simulink model "M4B11_modified_AGC_PI"  (R2025a)
settings: Solver=VariableStepAuto  StartTime=0.0  StopTime=100  RelTol=1e-3
InitFcn:
  | clear;
  | load('parameterinit.mat');
  | set_param('M4B11_modified_AGC_PI/Python2Sim','value','[0 0 0 0 0 0 0 0]');
  | acom=100;
  | bcom=50;
  | lam=100;
values from neighbouring files (symbols this model uses):
  ACgirdinit =     [datainit.mat]    (also in parameterinit.mat)
  AVm0 = [11.3576294988 11.3576294988]    [datainit.mat]    (also in parameterinit.mat)
  commun = [1 1 1 0]    [datainit.mat]    (also in initAll.m = [1,1,1,0]; parameterinit.mat)
  DataDelay = [0  0; 0  0; 0  0; 0  0]    [datainit.mat]    (also in initAll.m = 0.0*DataDelay; parameterinit.mat)
  ESinit =     [datainit.mat]    (also in parameterinit.mat)
  fB = 50    [datainit.mat]    (also in initAll.m; parameterinit.mat)
  Geninit =     [datainit.mat]    (also in initAll.m = Generator_init(opdata,SynMach_in_gidx); parameterinit.mat)
  SgridB = 100    [datainit.mat]    (also in initAll.m = resultsac.baseMVA; parameterinit.mat)
  wB = 314.159265359    [datainit.mat]    (also in initAll.m; parameterinit.mat)
  Windinit =     [datainit.mat]    (also in parameterinit.mat)
undefined symbols (not defined in the file or in its folder): c1, c2, c3, c4, c5, c6, cp_nom, lambda_nom, P_wind_base, Pelec_base, Pnom
libraries: spsBistableLib x9, slpidlib x2, simulink_extras x2
(part 5 of 6)

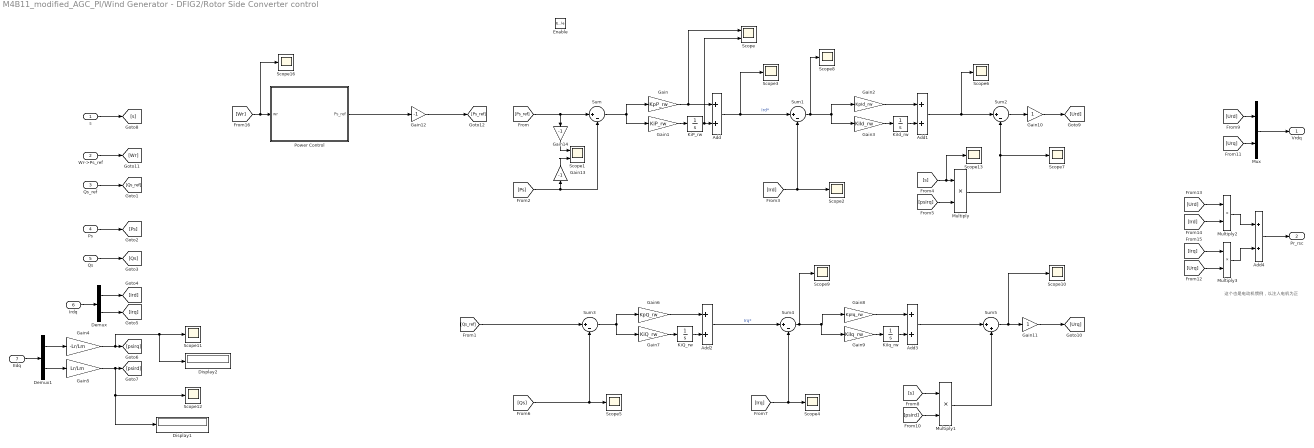
== system M4B11_modified_AGC_PI/Wind Generator - DFIG2/Rotor Side Converter control ==
  note: 这个也是电动机惯例，以注入电机为正
  s : Inport
  Wr->Ps_ref : Inport  Port=2
  Qs_ref : Inport  Port=3
  Ps : Inport  Port=4
  Qs : Inport  Port=5
  Irdq : Inport  Port=6
  Edq : Inport  Port=7
  Enable : EnablePort
  Add{,1..4} (5 alike) : Sum
  Demux : Demux  Outputs=2
  Demux1 : Demux  Outputs=2
  Display1 : Display
  Display2 : Display
  Gain : Gain  Gain=KpP_rw
  Gain1 : Gain  Gain=KiP_rw
  Gain10 : Gain
  Gain11 : Gain
  Gain12 : Gain  Gain=-1
  Gain13 : Gain  Gain=-1
  Gain14 : Gain  Gain=-1
  Gain2 : Gain  Gain=KpId_rw
  Gain3 : Gain  Gain=KiId_rw
  Gain4 : Gain  Gain=-Lr/Lm
  Gain5 : Gain  Gain=Lr/Lm
  Gain6 : Gain  Gain=KpQ_rw
  Gain7 : Gain  Gain=KiQ_rw
  Gain8 : Gain  Gain=KpIq_rw
  Gain9 : Gain  Gain=KiIq_rw
  KiId_rw : Integrator
  KiIq_rw : Integrator
  KiP_rw : Integrator  InitialCondition=Ird_ref
  KiQ_rw : Integrator  InitialCondition=Irq_ref
  Multiply{,1..3} (4 alike) : Product
  Mux : Mux  Inputs=2
  Power Control : Subsystem
  Scope : Scope  NumInputPorts=2
      settings: ActiveDisplayYMinimum=-0.15787  ActiveDisplayYMaximum=1.4048
  Scope1 : Scope  NumInputPorts=2
      settings: ActiveDisplayYMinimum=0.941157  ActiveDisplayYMaximum=0.94124  DataLoggingVariableName=ScopeData2
  Scope{2..13,16} (13 alike) : Scope
      Scope10 settings: ActiveDisplayYMinimum=-0.02713  ActiveDisplayYMaximum=0.00724  DataLoggingVariableName=ScopeData10
      Scope11 settings: DataLoggingVariableName=ScopeData13
      Scope12 settings: DataLoggingVariableName=ScopeData14
      Scope13 settings: ActiveDisplayYMinimum=-0.23407  ActiveDisplayYMaximum=0.19201  DataLoggingVariableName=ScopeData15
      Scope16 settings: ActiveDisplayYMinimum=-1.125  ActiveDisplayYMaximum=0.125  DataLoggingVariableName=ScopeData2
      Scope2 settings: ActiveDisplayYMinimum=0.9164  ActiveDisplayYMaximum=0.98721  DataLoggingVariableName=ScopeData4
      Scope3 settings: ActiveDisplayYMinimum=1.1610912356  ActiveDisplayYMaximum=1.1610912369  DataLoggingVariableName=ScopeData5
      Scope4 settings: ActiveDisplayYMinimum=-0.86275  ActiveDisplayYMaximum=6.60838  DataLoggingVariableName=ScopeData2
      Scope5 settings: ActiveDisplayYMinimum=-8E-13  ActiveDisplayYMaximum=6E-13  DataLoggingVariableName=ScopeData3
      Scope6 settings: ActiveDisplayYMinimum=0.00428  ActiveDisplayYMaximum=0.05974  DataLoggingVariableName=ScopeData2
      Scope7 settings: ActiveDisplayYMinimum=-0.10258  ActiveDisplayYMaximum=-0.10236  DataLoggingVariableName=ScopeData3
      Scope8 settings: ActiveDisplayYMinimum=-0.15319  ActiveDisplayYMaximum=1.32201  DataLoggingVariableName=ScopeData4
      Scope9 settings: ActiveDisplayYMinimum=-0.42548  ActiveDisplayYMaximum=0.04779  DataLoggingVariableName=ScopeData9
  Sum{,1..4} (5 alike) : Sum  Inputs=|+-
  Sum5 : Sum  Inputs=|++
  Vrdq : Outport
  Pr_rsc : Outport  Port=2
  wires:
  Gain12/1 -> [Ps_ref]
  Gain13/1 -> Scope1/2
  Gain14/1 -> Scope1/1
  [Qs_ref] -> Sum3/1
  Power Control/1(Ps_ref) -> Gain12/1
  [Wr] -> Power Control/1(wr), Scope16/1
  [Ird] -> Sum1/2, Scope2/1
  Add4/1 -> Pr_rsc/1
  Multiply3/1 -> Add4/2
  Multiply2/1 -> Add4/1
  [Urq] -> Multiply3/2
  [Irq] -> Multiply3/1
  [Ird] -> Multiply2/2
  [Urd] -> Multiply2/1
  KiP_rw/1 -> Add/2, Scope/2
  Gain/1 -> Add/1, Scope/1
  Gain11/1 -> [Urq]
  Gain10/1 -> [Urd]
  Mux/1 -> Vrdq/1
  [Urq] -> Mux/2
  [Urd] -> Mux/1
  Sum5/1 -> Gain11/1, Scope10/1
  Multiply1/1 -> Sum5/2
  [psird] -> Multiply1/2
  [s] -> Multiply1/1
  Add3/1 -> Sum5/1
  Gain9/1 -> KiIq_rw/1
  Sum4/1 -> Gain8/1, Gain9/1, Scope9/1
  Gain8/1 -> Add3/1
  KiIq_rw/1 -> Add3/2
  [Irq] -> Sum4/2, Scope4/1
  Gain7/1 -> KiQ_rw/1
  KiQ_rw/1 -> Add2/2
  Gain6/1 -> Add2/1
  Sum3/1 -> Gain6/1, Gain7/1
  Add2/1 -> Sum4/1  "Irq*"
  [Qs] -> Sum3/2, Scope5/1
  Sum2/1 -> Gain10/1
  Multiply/1 -> Sum2/2, Scope7/1
  [psirq] -> Multiply/2
  [s] -> Multiply/1, Scope13/1
  Gain5/1 -> [psird], Display1/1, Scope12/1
  Gain4/1 -> [psirq], Scope11/1, Display2/1
  Demux1/1 -> Gain4/1
  s/1 -> [s]
  Edq/1 -> Demux1/1
  Demux1/2 -> Gain5/1
  Gain3/1 -> KiId_rw/1
  KiId_rw/1 -> Add1/2
  Gain2/1 -> Add1/1
  Sum1/1 -> Gain2/1, Gain3/1, Scope8/1
  Add1/1 -> Sum2/1, Scope6/1
  Add/1 -> Scope3/1, Sum1/1  "Ird*"
  Sum/1 -> Gain/1, Gain1/1
  Gain1/1 -> KiP_rw/1
  [Ps] -> Gain13/1, Sum/2
  [Ps_ref] -> Sum/1, Gain14/1
  Demux/2 -> [Irq]
  Demux/1 -> [Ird]
  Irdq/1 -> Demux/1
  Qs/1 -> [Qs]
  Ps/1 -> [Ps]
  Qs_ref/1 -> [Qs_ref]
  Wr->Ps_ref/1 -> [Wr]

== system M4B11_modified_AGC_PI/Wind Generator - DFIG2/Wind Turbine ==
  note: $C_p=0.22* \lbrack 116*(\frac{1}{\lambda+0.008\beta}-\frac{0.0035}{\beta^3+1})-0.48\beta-5 \rbrack * e^{-12.5*(\frac{1}{\lambda+0.08\beta}-\frac{0.035}{\beta^3+1}) }$
  note: $P_m=0.95*\frac{1.2}{(12^3*0.5)}*\lbrack 43.268*(\frac{v_w}{99.4945*\omega_r}-0.035)-1.865 \rbrack * e^{-12.5*(\frac{v_w}{99.4945*\omega_r}-0.035) }*v_w^3$
  note: $C_p= \lbrack 43.268*(\frac{v_w}{99.4945*\omega_r}-0.035)-1.865 \rbrack * e^{-12.5*(\frac{v_w}{99.4945*\omega_r}-0.035) }$
  note: $P_m=0.95*\frac{1.2}{(12^3*0.5)}*\lbrack 43.268*(\frac{1}{99.4945*\frac{\omega_r}{v_w}}-0.035)-1.865 \rbrack * e^{-12.5*(\frac{1}{99.4945*\frac{\omega_r}{v_w}}-0.035) }*v_w^3$
  note: $C_p= \lbrack 43.268*(\frac{1}{99.4945*\frac{\omega_r}{v_w}}-0.035)-1.865 \rbrack * e^{-12.5*(\frac{1}{99.4945*\frac{\omega_r}{v_w}}-0.035) }$
  note: $P_m=0.95*\frac{1.2}{(12^3*0.5)}*C_p*v_w^3$
  note: $C_p= \lbrack 43.268*(\frac{1}{\lambda}-0.035)-1.865 \rbrack * e^{-12.5*(\frac{1}{\lambda}-0.035) }$
  note: $C_p=0.373* \lbrack 116*(\frac{1}{\lambda}-0.035)-5 \rbrack * e^{-12.5*(\frac{1}{\lambda}-0.035) }$
  note: 叶片旋转角速度
  note: 风力机输出
      | 的机械功率
  note: 叶尖速比
  note: 风能利用系数与桨矩角
      | 和叶尖速比之间的关系
  note: 风能利用
      | 系数
  note: 风力机输出
      | 的机械功率
  note: 风速
  note: 叶片旋转速度
  note: 考虑了机械损耗
  note: $\lambda=99.4945*\frac{\omega_r}{v_w}$
  note: $C_p=0.373* \lbrack 116*(\frac{1}{\lambda+0.08\beta}-\frac{0.035}{\beta^3+1})-0.4\beta-5 \rbrack * e^{-12.5*(\frac{1}{\lambda+0.08\beta}-\frac{0.035}{\beta^3+1}) }$
  note: $P_m=\frac{1.2}{(12^3*0.5)}*C_p*v_w^3$
  note: J. Chen and D. Jiang, "Study on modeling and simulation of non-grid-connected wind turbine," 2009 World Non-Grid-Connected Wind Power and Energy Conference , Nanjing, 2009, pp. 1-5. doi: 10.1109/WNWEC.2009.5335791
  W_wt (pu) : Inport
  Pitch angle (deg) : Inport  Port=2
  Wind speed (m/s) : Inport  Port=3
  ->pu1 : Gain  Gain=0.95
  ->pu2 : Gain  Gain=0.95
  Avoid div. by zero : Saturate  UpperLimit=inf  LowerLimit=eps
  "Avoid div. by zero " : Saturate  UpperLimit=inf  LowerLimit=eps
  Display2 : Display
  Fcn2 : Fcn  Expr=99.4945*u[2]/u[1]
  Fcn4 : Fcn  Expr=0.22*(116*(1/(u(1)+0.008*u(2))-0.0035/((u(2)^3)+1))-0.48*u(2)-5)*exp(-12.5*(1/(u(1)+0.008*u(2))-0.0035/((u(2)^3)+1)))
  "K2*Cp*wind^3 " : Fcn  Expr=1.2/(12^3*0.5)*u[1]^3*u[2]
  Mux : Mux  Inputs=2
  Mux1 : Mux  Inputs=2
  Mux2 : Mux  Inputs=2
  Product2 : Product  Inputs=*/  InputSameDT=on  SaturateOnIntegerOverflow=on  OutDataTypeStr=Inherit: Same as first input
  Scope{1..3,5} (4 alike) : Scope
      Scope1 settings: ActiveDisplayYMinimum=6.3327  ActiveDisplayYMaximum=6.33385  DataLoggingSaveFormat=Array
      Scope2 settings: ActiveDisplayYMinimum=0.10425  ActiveDisplayYMaximum=1.46932  DataLoggingVariableName=ScopeData25
      Scope3 settings: ActiveDisplayYMinimum=0.5999  ActiveDisplayYMaximum=0.6001  DataLoggingVariableName=Pw  DataLoggingSaveFormat=Array
      Scope5 settings: ActiveDisplayYMinimum=0.64296  ActiveDisplayYMaximum=0.84296  DataLoggingVariableName=Pw2  DataLoggingSaveFormat=Array
  Subsystem : Subsystem  Commented=on
  Tm : Outport
  Pm : Outport  Port=2
  wires:
  ->pu2/1 -> Pm/1
  Fcn4/1 -> Scope5/1, Mux2/2
  "K2*Cp*wind^3 "/1 -> Scope3/1, Display2/1, Product2/1, ->pu2/1
  Wind speed (m/s)/1 -> Avoid div. by zero/1
  Product2/1 -> ->pu1/1
  ->pu1/1 -> Scope2/1, Tm/1
  W_wt (pu)/1 -> "Avoid div. by zero "/1
  "Avoid div. by zero "/1 -> Product2/2, Mux/2
  Avoid div. by zero/1 -> Mux2/1, Mux/1
  Pitch angle (deg)/1 -> Mux1/2
  Mux2/1 -> "K2*Cp*wind^3 "/1
  Mux/1 -> Fcn2/1
  Mux1/1 -> Fcn4/1
  Fcn2/1 -> Mux1/1, Scope1/1  "lambda"

== system M4B11_modified_AGC_PI/Wind Generator - DFIG2/dq-xy ==
  dq : Inport
  delta_xy : Inport  Port=2
  Complex to Magnitude-Angle : ComplexToMagnitudeAngle
  Demux : Demux  Outputs=2
  Fcn3 : Fcn  Expr=u(1)*cos(u(2))
  Fcn4 : Fcn  Expr=u(1)*sin(u(2))
  Mux1 : Mux  Inputs=2
  Mux2 : Mux  Inputs=2
  Real-Imag to Complex : RealImagToComplex
  Scope : Scope
      settings: ActiveDisplayYMinimum=0.298155365983  ActiveDisplayYMaximum=0.298155366015  DataLoggingVariableName=ScopeData2
  Scope1 : Scope  NumInputPorts=2
      settings: ActiveDisplayYMinimum=1.04058  ActiveDisplayYMaximum=1.12593  DataLoggingVariableName=ScopeData51  DataLoggingSaveFormat=Array
  Scope2 : Scope  NumInputPorts=2
      settings: ActiveDisplayYMinimum=1.01502  ActiveDisplayYMaximum=1.10979  DataLoggingVariableName=ScopeData56  DataLoggingSaveFormat=Array
  Sum14 : Sum  Inputs=|++
  xy : Outport
  wires:
  Mux2/1 -> xy/1
  dq/1 -> Demux/1
  Demux/2 -> Real-Imag to Complex/2
  Demux/1 -> Real-Imag to Complex/1
  Real-Imag to Complex/1 -> Complex to Magnitude-Angle/1
  delta_xy/1 -> Sum14/2
  Fcn3/1 -> Mux2/1, Scope2/1
  Fcn4/1 -> Scope2/2, Mux2/2
  Mux1/1 -> Fcn3/1, Fcn4/1
  Complex to Magnitude-Angle/2 -> Sum14/1, Scope/1
  Complex to Magnitude-Angle/1 -> Mux1/1, Scope1/1
  Sum14/1 -> Mux1/2, Scope1/2

== system M4B11_modified_AGC_PI/Wind Generator - DFIG2/dq-xy1 ==
  dq : Inport
  delta_xy : Inport  Port=2
  Complex to Magnitude-Angle : ComplexToMagnitudeAngle
  Demux : Demux  Outputs=2
  Fcn3 : Fcn  Expr=u(1)*cos(u(2))
  Fcn4 : Fcn  Expr=u(1)*sin(u(2))
  Mux1 : Mux  Inputs=2
  Mux2 : Mux  Inputs=2
  Real-Imag to Complex : RealImagToComplex
  Scope : Scope
      settings: ActiveDisplayYMinimum=0.298155365983  ActiveDisplayYMaximum=0.298155366015  DataLoggingVariableName=ScopeData2
  Scope1 : Scope  NumInputPorts=2
      settings: ActiveDisplayYMinimum=1.04058  ActiveDisplayYMaximum=1.12593  DataLoggingVariableName=ScopeData51  DataLoggingSaveFormat=Array
  Scope2 : Scope  NumInputPorts=2
      settings: ActiveDisplayYMinimum=1.01502  ActiveDisplayYMaximum=1.10979  DataLoggingVariableName=ScopeData56  DataLoggingSaveFormat=Array
  Sum14 : Sum  Inputs=|++
  xy : Outport
  wires:
  Mux2/1 -> xy/1
  dq/1 -> Demux/1
  Demux/2 -> Real-Imag to Complex/2
  Demux/1 -> Real-Imag to Complex/1
  Real-Imag to Complex/1 -> Complex to Magnitude-Angle/1
  delta_xy/1 -> Sum14/2
  Fcn3/1 -> Mux2/1, Scope2/1
  Fcn4/1 -> Scope2/2, Mux2/2
  Mux1/1 -> Fcn3/1, Fcn4/1
  Complex to Magnitude-Angle/2 -> Sum14/1, Scope/1
  Complex to Magnitude-Angle/1 -> Mux1/1, Scope1/1
  Sum14/1 -> Mux1/2, Scope1/2

== system M4B11_modified_AGC_PI/Wind Generator - DFIG2/help ==
  note: $P_m=0.95*\frac{1.2}{(12^3*0.5)}*\lbrack 43.268*(\frac{v_w}{99.4945*\omega_r}-0.035)-1.865 \rbrack * e^{-12.5*(\frac{v_w}{99.4945*\omega_r}-0.035) }*v_w^3$
  note: $P_w=P_m=(1-s)*P_s=\omega_r*2*(0.5*\omega_r^2+0.05*\omega_r+0.12)$
  note: $P_s^{ref}=2*(0.5000*\omega_r^2+0.0500*\omega_r+0.1200)$
  note: 从诺顿支路的角度考虑，VSC可以等效成纯的电流源，与等效成诺顿支路的异步电机的虚拟电流应该是可以直接相加
      | 现在关键问题是，异步电机的虚拟电流已经转换成了xy坐标系下的量。
      | 我下面要证明
      | 异步电机实际电流Igxy+VSC实际电流Icxy= [（异步电机实际电流Igdq+VSC实际电流Icdq）-->xy]
  note: $I_{gxy}+I_{cxy}\\ =[-I_{gxy}^{\prime}+(ZP)^{-1}PV_{gxy}]+I_{cxy}$
  note: $-I_{sdq}=I_{sdq}^{\prime}-Z^{-1}V_{sdq}\\ 其中I_{sdq}^{\prime}=Z^{-1}E_{dq}$
  note: 可以看到完全一致，在模型中可以先变Icdq为Icxy，再与虚拟电流xy相加
  note: $I_{gxy}+I_{cxy}\\ =[-I_{gxy}^{\prime}+(ZP)^{-1}PV_{gxy}]+I_{cxy}$
  note: $PV_{sxy}=E_{dq}+ZPI_{sxy}$
  note: $\pmatrix{A_d \cr A_q}=\pmatrix{cos\theta & sin\theta \cr -sin\theta & cos\theta}\pmatrix{A_x \cr A_y}\\ P=\pmatrix{cos\theta & sin\theta \cr -sin\theta & cos\theta}$
  note: $(ZP)^{-1}PV_{sxy}=(ZP)^{-1}E_{dq}+I_{sxy}$
  note: $-I_{sxy}=(ZP)^{-1}E_{dq}-(ZP)^{-1}PV_{sxy}$
  note: $A_{dq}=PA_{xy}\\ A_{xy}=P^{-1}A_{dq}$
  note: $-I_{sxy}=I_{sxy}^{\prime}-(ZP)^{-1}PV_{sxy}\\ 其中I_{sxy}^{\prime}=(ZP)^{-1}E_{dq}$
  note: $V_{sdq}=E_{dq}+ZI_{sdq}$
  note: $-I_{sdq}=Z^{-1}E_{dq}-Z^{-1}V_{sdq}$
  note: $V_{sdq}=E_{dq}+ZI_{sdq}$
  note: $PI_{gxy}+PI_{cxy}\\ =[-PI_{gxy}^{\prime}+Z^{-1}PV_{gxy}]+PI_{cxy}$
  note: $I_{gxy}+I_{cxy}\\ =[-I_{gxy}^{\prime}+P^{-1}Z^{-1}PV_{gxy}]+I_{cxy}$
  note: $I_{gdq}+I_{cdq}\\ =[-I_{gdq}^{\prime}+Z^{-1}V_{gdq}]+I_{cdq}$
  note: $Z^{-1}V_{sdq}=Z^{-1}E_{dq}+I_{sdq}$
  note: $\omega_{r}=(1-s)*\omega_1$

== system M4B11_modified_AGC_PI/Wind Generator - DFIG2/output ==
  Isxy1 : Inport
  Ixy_gsc : Inport  Port=2
  GB : Inport  Port=3
  Ps : Inport  Port=4
  Prgsc : Inport  Port=5
  fw : Inport  Port=6
  Wr : Inport  Port=7
  Add : Sum
  Add1 : Sum
  Bus Creator : BusCreator  Inputs=3
  Demux : Demux
  Gain2 : Gain  Gain=SwgeqB./SgridB
  Gain3 : Gain
  Gain4 : Gain
  Gain5 : Gain  Gain=-1
  Gain6 : Gain  Gain=SwgeqB./SgridB
  Gain7 : Gain  Gain=-1
  Gain8 : Gain  Gain=SwgeqB./SgridB
  Scope : Scope  NumInputPorts=4
      settings: ActiveDisplayYMinimum=-54.46215  ActiveDisplayYMaximum=-34.46215  DataLoggingVariableName=ScopeData5
  Scope{4..5,7..8} (4 alike) : Scope
      Scope4 settings: ActiveDisplayYMinimum=-50.97357  ActiveDisplayYMaximum=11.3279  DataLoggingVariableName=ScopeData4
      Scope5 settings: TimeSpan=200  ActiveDisplayYMinimum=0.47861  ActiveDisplayYMaximum=6.19543  DataLoggingVariableName=ScopeData6
      Scope7 settings: ActiveDisplayYMinimum=-2.00383  ActiveDisplayYMaximum=-0.83205  DataLoggingVariableName=ScopeData7
      Scope8 settings: ActiveDisplayYMinimum=-0.15764  ActiveDisplayYMaximum=0.7029  DataLoggingVariableName=ScopeData8
  m : Outport
  Igxy : Outport  Port=2
  GBxy : Outport  Port=3
  wires:
  Wr/1 -> Bus Creator/3  "Wr"
  fw/1 -> Bus Creator/2  "fw"
  Bus Creator/1 -> m/1
  Ps/1 -> Add1/1, Scope7/1
  Add1/1 -> Gain7/1
  Gain7/1 -> Gain8/1
  Gain8/1 -> Bus Creator/1, Scope5/1  "Pwind"
  Prgsc/1 -> Add1/2, Scope8/1
  GB/1 -> Gain3/1
  Gain3/1 -> Gain6/1
  Gain6/1 -> GBxy/1, Demux/1
  Demux/3 -> Scope/3
  Demux/4 -> Scope/4
  Demux/1 -> Scope/1
  Demux/2 -> Scope/2
  Gain5/1 -> Add/2
  Gain4/1 -> Add/1
  Ixy_gsc/1 -> Gain5/1
  Add/1 -> Gain2/1
  Gain2/1 -> Scope4/1, Igxy/1
  Isxy1/1 -> Gain4/1

== system M4B11_modified_AGC_PI/Wind Generator - DFIG2/xy->dq1 ==
  Ixy : Inport
  Theta : Inport  Port=2
  Complex to Magnitude-Angle : ComplexToMagnitudeAngle
  Complex to Real-Imag : ComplexToRealImag
  Demux1 : Demux  Outputs=2
      settings: DisplayOption=none
  Magnitude-Angle to Complex : MagnitudeAngleToComplex
  Mux : Mux  Inputs=2
  Real-Imag to Complex : RealImagToComplex
  Scope : Scope
      settings: ActiveDisplayYMinimum=3.11918  ActiveDisplayYMaximum=3.16079
  Scope1 : Scope
      settings: ActiveDisplayYMinimum=2.59405  ActiveDisplayYMaximum=3.13201  DataLoggingVariableName=ScopeData3
  Sum1 : Sum  Inputs=|+-  SaturateOnIntegerOverflow=on
  Idq : Outport
  wires:
  Complex to Magnitude-Angle/1 -> Magnitude-Angle to Complex/1
  Theta/1 -> Sum1/2
  Complex to Magnitude-Angle/2 -> Sum1/1, Scope1/1
  Demux1/1 -> Real-Imag to Complex/1
  Complex to Real-Imag/2 -> Mux/2  "Iq"
  Mux/1 -> Idq/1
  Complex to Real-Imag/1 -> Mux/1  "Id"
  Magnitude-Angle to Complex/1 -> Complex to Real-Imag/1
  Sum1/1 -> Magnitude-Angle to Complex/2, Scope/1
  Demux1/2 -> Real-Imag to Complex/2
  Real-Imag to Complex/1 -> Complex to Magnitude-Angle/1
  Ixy/1 -> Demux1/1

== system M4B11_modified_AGC_PI/Wind Generator - DFIG2/xy->dq2 ==
  Ixy : Inport
  Theta : Inport  Port=2
  Complex to Magnitude-Angle : ComplexToMagnitudeAngle
  Complex to Real-Imag : ComplexToRealImag
  Demux1 : Demux  Outputs=2
      settings: DisplayOption=none
  Magnitude-Angle to Complex : MagnitudeAngleToComplex
  Mux : Mux  Inputs=2
  Real-Imag to Complex : RealImagToComplex
  Scope : Scope
      settings: ActiveDisplayYMinimum=3.11918  ActiveDisplayYMaximum=3.16079
  Scope1 : Scope
      settings: ActiveDisplayYMinimum=2.59405  ActiveDisplayYMaximum=3.13201  DataLoggingVariableName=ScopeData3
  Sum1 : Sum  Inputs=|+-  SaturateOnIntegerOverflow=on
  Idq : Outport
  wires:
  Complex to Magnitude-Angle/1 -> Magnitude-Angle to Complex/1
  Theta/1 -> Sum1/2
  Complex to Magnitude-Angle/2 -> Sum1/1, Scope1/1
  Demux1/1 -> Real-Imag to Complex/1
  Complex to Real-Imag/2 -> Mux/2  "Iq"
  Mux/1 -> Idq/1
  Complex to Real-Imag/1 -> Mux/1  "Id"
  Magnitude-Angle to Complex/1 -> Complex to Real-Imag/1
  Sum1/1 -> Magnitude-Angle to Complex/2, Scope/1
  Demux1/2 -> Real-Imag to Complex/2
  Real-Imag to Complex/1 -> Complex to Magnitude-Angle/1
  Ixy/1 -> Demux1/1

== system M4B11_modified_AGC_PI/Wind Generator - DFIG2/xy->dq3 ==
  Ixy : Inport
  Theta : Inport  Port=2
  Complex to Magnitude-Angle : ComplexToMagnitudeAngle
  Complex to Real-Imag : ComplexToRealImag
  Demux1 : Demux  Outputs=2
      settings: DisplayOption=none
  Magnitude-Angle to Complex : MagnitudeAngleToComplex
  Mux : Mux  Inputs=2
  Real-Imag to Complex : RealImagToComplex
  Scope : Scope
      settings: ActiveDisplayYMinimum=3.11918  ActiveDisplayYMaximum=3.16079
  Scope1 : Scope
      settings: ActiveDisplayYMinimum=2.59405  ActiveDisplayYMaximum=3.13201  DataLoggingVariableName=ScopeData3
  Sum1 : Sum  Inputs=|+-  SaturateOnIntegerOverflow=on
  Idq : Outport
  wires:
  Complex to Magnitude-Angle/1 -> Magnitude-Angle to Complex/1
  Theta/1 -> Sum1/2
  Complex to Magnitude-Angle/2 -> Sum1/1, Scope1/1
  Demux1/1 -> Real-Imag to Complex/1
  Complex to Real-Imag/2 -> Mux/2  "Iq"
  Mux/1 -> Idq/1
  Complex to Real-Imag/1 -> Mux/1  "Id"
  Magnitude-Angle to Complex/1 -> Complex to Real-Imag/1
  Sum1/1 -> Magnitude-Angle to Complex/2, Scope/1
  Demux1/2 -> Real-Imag to Complex/2
  Real-Imag to Complex/1 -> Complex to Magnitude-Angle/1
  Ixy/1 -> Demux1/1

== system M4B11_modified_AGC_PI/ES1/ control1/control_AC_voltage ==
  usd : Inport
  usdref : Inport  Port=2
  Out_Q_Uac : Subsystem  mask{KP_=Kpac_VSC_A, KI_=Kiac_VSC_A, Upper_limit=inf, Lower_limit=-inf, Upper_saturation_limit=inf, Lower_saturation_limit=-inf, integrator_init=Nd_A_0}
      mask prompts: KP_ "比例系数P"; KI_ "积分系数I"; Upper_limit "限幅上限"; Lower_limit "限幅下限"; Upper_saturation_limit "积分饱和上限"; Lower_saturation_limit "积分饱和下限"; integrator_init "积分初始值"
      mask DialogControl Container4 Prompt: 控制参数
      mask DialogControl Container5 Prompt: 初始值
      mask Display: disp('PI')
  Scope : Scope  NumInputPorts=2
      settings: ActiveDisplayYMinimum=1.00888  ActiveDisplayYMaximum=1.01608  DataLoggingVariableName=ScopeData3
  Sum13 : Sum  Inputs=|+-  SaturateOnIntegerOverflow=on
  isdref : Outport
  wires:
  Sum13/1 -> Out_Q_Uac/1(In1)
  Out_Q_Uac/1(Out1) -> isdref/1
  usd/1 -> Scope/2, Sum13/1
  usdref/1 -> Scope/1, Sum13/2

== system M4B11_modified_AGC_PI/ES1/ control1/control_AC_voltage1 ==
  usq : Inport
  usqref : Inport  Port=2
  Out_Q_Uac : Subsystem  mask{KP_=Kpac_VSC_A, KI_=Kiac_VSC_A, Upper_limit=inf, Lower_limit=-inf, Upper_saturation_limit=inf, Lower_saturation_limit=-inf, integrator_init=Nq_A_0}
      mask prompts: KP_ "比例系数P"; KI_ "积分系数I"; Upper_limit "限幅上限"; Lower_limit "限幅下限"; Upper_saturation_limit "积分饱和上限"; Lower_saturation_limit "积分饱和下限"; integrator_init "积分初始值"
      mask DialogControl Container4 Prompt: 控制参数
      mask DialogControl Container5 Prompt: 初始值
      mask Display: disp('PI')
  Sum13 : Sum  Inputs=|+-  SaturateOnIntegerOverflow=on
  isqref : Outport
  wires:
  Sum13/1 -> Out_Q_Uac/1(In1)
  Out_Q_Uac/1(Out1) -> isqref/1
  usqref/1 -> Sum13/2
  usq/1 -> Sum13/1

== system M4B11_modified_AGC_PI/ES1/ control1/in_D_PI ==
  In1 : Inport
  Ki : Gain  Gain=KI_  SaturateOnIntegerOverflow=on  OutDataTypeStr=Inherit: Same as input  ParamDataTypeStr=Inherit: Same as input
  Kp : Gain  Gain=KP_  SaturateOnIntegerOverflow=on  OutDataTypeStr=Inherit: Same as input  ParamDataTypeStr=Inherit: Same as input
  Saturation2 : Saturate  UpperLimit=Upper_limit  LowerLimit=Lower_limit
  Sum12 : Sum  SaturateOnIntegerOverflow=on
  integrator : Integrator  InitialCondition=integrator_init  LimitOutput=on  UpperSaturationLimit=Upper_saturation_limit  LowerSaturationLimit=Lower_saturation_limit
  Out1 : Outport
  wires:
  In1/1 -> Ki/1, Kp/1
  Kp/1 -> Sum12/2
  Ki/1 -> integrator/1
  integrator/1 -> Sum12/1
  Saturation2/1 -> Out1/1
  Sum12/1 -> Saturation2/1

== system M4B11_modified_AGC_PI/ES1/ control1/in_Q_PI ==
  In1 : Inport
  Ki : Gain  Gain=KI_  SaturateOnIntegerOverflow=on  OutDataTypeStr=Inherit: Same as input  ParamDataTypeStr=Inherit: Same as input
  Kp : Gain  Gain=KP_  SaturateOnIntegerOverflow=on  OutDataTypeStr=Inherit: Same as input  ParamDataTypeStr=Inherit: Same as input
  Saturation2 : Saturate  UpperLimit=Upper_limit  LowerLimit=Lower_limit
  Sum12 : Sum  SaturateOnIntegerOverflow=on
  integrator : Integrator  InitialCondition=integrator_init  LimitOutput=on  UpperSaturationLimit=Upper_saturation_limit  LowerSaturationLimit=Lower_saturation_limit
  Out1 : Outport
  wires:
  In1/1 -> Ki/1, Kp/1
  Kp/1 -> Sum12/2
  Ki/1 -> integrator/1
  integrator/1 -> Sum12/1
  Saturation2/1 -> Out1/1
  Sum12/1 -> Saturation2/1

== system M4B11_modified_AGC_PI/ES2/ control1/control_AC_voltage ==
  usd : Inport
  usdref : Inport  Port=2
  Out_Q_Uac : Subsystem  mask{KP_=Kpac_VSC_A, KI_=Kiac_VSC_A, Upper_limit=inf, Lower_limit=-inf, Upper_saturation_limit=inf, Lower_saturation_limit=-inf, integrator_init=Nd_A_0}
      mask prompts: KP_ "比例系数P"; KI_ "积分系数I"; Upper_limit "限幅上限"; Lower_limit "限幅下限"; Upper_saturation_limit "积分饱和上限"; Lower_saturation_limit "积分饱和下限"; integrator_init "积分初始值"
      mask DialogControl Container4 Prompt: 控制参数
      mask DialogControl Container5 Prompt: 初始值
      mask Display: disp('PI')
  Sum13 : Sum  Inputs=|+-  SaturateOnIntegerOverflow=on
  isdref : Outport
  wires:
  Sum13/1 -> Out_Q_Uac/1(In1)
  Out_Q_Uac/1(Out1) -> isdref/1
  usdref/1 -> Sum13/2
  usd/1 -> Sum13/1

== system M4B11_modified_AGC_PI/ES2/ control1/control_AC_voltage1 ==
  usq : Inport
  usqref : Inport  Port=2
  Out_Q_Uac : Subsystem  mask{KP_=Kpac_VSC_A, KI_=Kiac_VSC_A, Upper_limit=inf, Lower_limit=-inf, Upper_saturation_limit=inf, Lower_saturation_limit=-inf, integrator_init=Nq_A_0}
      mask prompts: KP_ "比例系数P"; KI_ "积分系数I"; Upper_limit "限幅上限"; Lower_limit "限幅下限"; Upper_saturation_limit "积分饱和上限"; Lower_saturation_limit "积分饱和下限"; integrator_init "积分初始值"
      mask DialogControl Container4 Prompt: 控制参数
      mask DialogControl Container5 Prompt: 初始值
      mask Display: disp('PI')
  Sum13 : Sum  Inputs=|+-  SaturateOnIntegerOverflow=on
  isqref : Outport
  wires:
  Sum13/1 -> Out_Q_Uac/1(In1)
  Out_Q_Uac/1(Out1) -> isqref/1
  usqref/1 -> Sum13/2
  usq/1 -> Sum13/1

== system M4B11_modified_AGC_PI/ES2/ control1/in_D_PI ==
  In1 : Inport
  Ki : Gain  Gain=KI_  SaturateOnIntegerOverflow=on  OutDataTypeStr=Inherit: Same as input  ParamDataTypeStr=Inherit: Same as input
  Kp : Gain  Gain=KP_  SaturateOnIntegerOverflow=on  OutDataTypeStr=Inherit: Same as input  ParamDataTypeStr=Inherit: Same as input
  Saturation2 : Saturate  UpperLimit=Upper_limit  LowerLimit=Lower_limit
  Sum12 : Sum  SaturateOnIntegerOverflow=on
  integrator : Integrator  InitialCondition=integrator_init  LimitOutput=on  UpperSaturationLimit=Upper_saturation_limit  LowerSaturationLimit=Lower_saturation_limit
  Out1 : Outport
  wires:
  In1/1 -> Ki/1, Kp/1
  Kp/1 -> Sum12/2
  Ki/1 -> integrator/1
  integrator/1 -> Sum12/1
  Saturation2/1 -> Out1/1
  Sum12/1 -> Saturation2/1

== system M4B11_modified_AGC_PI/ES2/ control1/in_Q_PI ==
  In1 : Inport
  Ki : Gain  Gain=KI_  SaturateOnIntegerOverflow=on  OutDataTypeStr=Inherit: Same as input  ParamDataTypeStr=Inherit: Same as input
  Kp : Gain  Gain=KP_  SaturateOnIntegerOverflow=on  OutDataTypeStr=Inherit: Same as input  ParamDataTypeStr=Inherit: Same as input
  Saturation2 : Saturate  UpperLimit=Upper_limit  LowerLimit=Lower_limit
  Sum12 : Sum  SaturateOnIntegerOverflow=on
  integrator : Integrator  InitialCondition=integrator_init  LimitOutput=on  UpperSaturationLimit=Upper_saturation_limit  LowerSaturationLimit=Lower_saturation_limit
  Out1 : Outport
  wires:
  In1/1 -> Ki/1, Kp/1
  Kp/1 -> Sum12/2
  Ki/1 -> integrator/1
  integrator/1 -> Sum12/1
  Saturation2/1 -> Out1/1
  Sum12/1 -> Saturation2/1

== system M4B11_modified_AGC_PI/ES3/ control1/control_AC_voltage ==
  usd : Inport
  usdref : Inport  Port=2
  Out_Q_Uac : Subsystem  mask{KP_=Kpac_VSC_A, KI_=Kiac_VSC_A, Upper_limit=inf, Lower_limit=-inf, Upper_saturation_limit=inf, Lower_saturation_limit=-inf, integrator_init=Nd_A_0}
      mask prompts: KP_ "比例系数P"; KI_ "积分系数I"; Upper_limit "限幅上限"; Lower_limit "限幅下限"; Upper_saturation_limit "积分饱和上限"; Lower_saturation_limit "积分饱和下限"; integrator_init "积分初始值"
      mask DialogControl Container4 Prompt: 控制参数
      mask DialogControl Container5 Prompt: 初始值
      mask Display: disp('PI')
  Sum13 : Sum  Inputs=|+-  SaturateOnIntegerOverflow=on
  isdref : Outport
  wires:
  Sum13/1 -> Out_Q_Uac/1(In1)
  Out_Q_Uac/1(Out1) -> isdref/1
  usdref/1 -> Sum13/2
  usd/1 -> Sum13/1

== system M4B11_modified_AGC_PI/ES3/ control1/control_AC_voltage1 ==
  usq : Inport
  usqref : Inport  Port=2
  Out_Q_Uac : Subsystem  mask{KP_=Kpac_VSC_A, KI_=Kiac_VSC_A, Upper_limit=inf, Lower_limit=-inf, Upper_saturation_limit=inf, Lower_saturation_limit=-inf, integrator_init=Nq_A_0}
      mask prompts: KP_ "比例系数P"; KI_ "积分系数I"; Upper_limit "限幅上限"; Lower_limit "限幅下限"; Upper_saturation_limit "积分饱和上限"; Lower_saturation_limit "积分饱和下限"; integrator_init "积分初始值"
      mask DialogControl Container4 Prompt: 控制参数
      mask DialogControl Container5 Prompt: 初始值
      mask Display: disp('PI')
  Sum13 : Sum  Inputs=|+-  SaturateOnIntegerOverflow=on
  isqref : Outport
  wires:
  Sum13/1 -> Out_Q_Uac/1(In1)
  Out_Q_Uac/1(Out1) -> isqref/1
  usqref/1 -> Sum13/2
  usq/1 -> Sum13/1

== system M4B11_modified_AGC_PI/ES3/ control1/in_D_PI ==
  In1 : Inport
  Ki : Gain  Gain=KI_  SaturateOnIntegerOverflow=on  OutDataTypeStr=Inherit: Same as input  ParamDataTypeStr=Inherit: Same as input
  Kp : Gain  Gain=KP_  SaturateOnIntegerOverflow=on  OutDataTypeStr=Inherit: Same as input  ParamDataTypeStr=Inherit: Same as input
  Saturation2 : Saturate  UpperLimit=Upper_limit  LowerLimit=Lower_limit
  Sum12 : Sum  SaturateOnIntegerOverflow=on
  integrator : Integrator  InitialCondition=integrator_init  LimitOutput=on  UpperSaturationLimit=Upper_saturation_limit  LowerSaturationLimit=Lower_saturation_limit
  Out1 : Outport
  wires:
  In1/1 -> Ki/1, Kp/1
  Kp/1 -> Sum12/2
  Ki/1 -> integrator/1
  integrator/1 -> Sum12/1
  Saturation2/1 -> Out1/1
  Sum12/1 -> Saturation2/1

== system M4B11_modified_AGC_PI/ES3/ control1/in_Q_PI ==
  In1 : Inport
  Ki : Gain  Gain=KI_  SaturateOnIntegerOverflow=on  OutDataTypeStr=Inherit: Same as input  ParamDataTypeStr=Inherit: Same as input
  Kp : Gain  Gain=KP_  SaturateOnIntegerOverflow=on  OutDataTypeStr=Inherit: Same as input  ParamDataTypeStr=Inherit: Same as input
  Saturation2 : Saturate  UpperLimit=Upper_limit  LowerLimit=Lower_limit
  Sum12 : Sum  SaturateOnIntegerOverflow=on
  integrator : Integrator  InitialCondition=integrator_init  LimitOutput=on  UpperSaturationLimit=Upper_saturation_limit  LowerSaturationLimit=Lower_saturation_limit
  Out1 : Outport
  wires:
  In1/1 -> Ki/1, Kp/1
  Kp/1 -> Sum12/2
  Ki/1 -> integrator/1
  integrator/1 -> Sum12/1
  Saturation2/1 -> Out1/1
  Sum12/1 -> Saturation2/1

== system M4B11_modified_AGC_PI/ES4/ control1/control_AC_voltage ==
  usd : Inport
  usdref : Inport  Port=2
  Out_Q_Uac : Subsystem  mask{KP_=Kpac_VSC_A, KI_=Kiac_VSC_A, Upper_limit=inf, Lower_limit=-inf, Upper_saturation_limit=inf, Lower_saturation_limit=-inf, integrator_init=Nd_A_0}
      mask prompts: KP_ "比例系数P"; KI_ "积分系数I"; Upper_limit "限幅上限"; Lower_limit "限幅下限"; Upper_saturation_limit "积分饱和上限"; Lower_saturation_limit "积分饱和下限"; integrator_init "积分初始值"
      mask DialogControl Container4 Prompt: 控制参数
      mask DialogControl Container5 Prompt: 初始值
      mask Display: disp('PI')
  Sum13 : Sum  Inputs=|+-  SaturateOnIntegerOverflow=on
  isdref : Outport
  wires:
  Sum13/1 -> Out_Q_Uac/1(In1)
  Out_Q_Uac/1(Out1) -> isdref/1
  usdref/1 -> Sum13/2
  usd/1 -> Sum13/1

== system M4B11_modified_AGC_PI/ES4/ control1/control_AC_voltage1 ==
  usq : Inport
  usqref : Inport  Port=2
  Out_Q_Uac : Subsystem  mask{KP_=Kpac_VSC_A, KI_=Kiac_VSC_A, Upper_limit=inf, Lower_limit=-inf, Upper_saturation_limit=inf, Lower_saturation_limit=-inf, integrator_init=Nq_A_0}
      mask prompts: KP_ "比例系数P"; KI_ "积分系数I"; Upper_limit "限幅上限"; Lower_limit "限幅下限"; Upper_saturation_limit "积分饱和上限"; Lower_saturation_limit "积分饱和下限"; integrator_init "积分初始值"
      mask DialogControl Container4 Prompt: 控制参数
      mask DialogControl Container5 Prompt: 初始值
      mask Display: disp('PI')
  Sum13 : Sum  Inputs=|+-  SaturateOnIntegerOverflow=on
  isqref : Outport
  wires:
  Sum13/1 -> Out_Q_Uac/1(In1)
  Out_Q_Uac/1(Out1) -> isqref/1
  usqref/1 -> Sum13/2
  usq/1 -> Sum13/1

== system M4B11_modified_AGC_PI/ES4/ control1/in_D_PI ==
  In1 : Inport
  Ki : Gain  Gain=KI_  SaturateOnIntegerOverflow=on  OutDataTypeStr=Inherit: Same as input  ParamDataTypeStr=Inherit: Same as input
  Kp : Gain  Gain=KP_  SaturateOnIntegerOverflow=on  OutDataTypeStr=Inherit: Same as input  ParamDataTypeStr=Inherit: Same as input
  Saturation2 : Saturate  UpperLimit=Upper_limit  LowerLimit=Lower_limit
  Sum12 : Sum  SaturateOnIntegerOverflow=on
  integrator : Integrator  InitialCondition=integrator_init  LimitOutput=on  UpperSaturationLimit=Upper_saturation_limit  LowerSaturationLimit=Lower_saturation_limit
  Out1 : Outport
  wires:
  In1/1 -> Ki/1, Kp/1
  Kp/1 -> Sum12/2
  Ki/1 -> integrator/1
  integrator/1 -> Sum12/1
  Saturation2/1 -> Out1/1
  Sum12/1 -> Saturation2/1

== system M4B11_modified_AGC_PI/ES4/ control1/in_Q_PI ==
  In1 : Inport
  Ki : Gain  Gain=KI_  SaturateOnIntegerOverflow=on  OutDataTypeStr=Inherit: Same as input  ParamDataTypeStr=Inherit: Same as input
  Kp : Gain  Gain=KP_  SaturateOnIntegerOverflow=on  OutDataTypeStr=Inherit: Same as input  ParamDataTypeStr=Inherit: Same as input
  Saturation2 : Saturate  UpperLimit=Upper_limit  LowerLimit=Lower_limit
  Sum12 : Sum  SaturateOnIntegerOverflow=on
  integrator : Integrator  InitialCondition=integrator_init  LimitOutput=on  UpperSaturationLimit=Upper_saturation_limit  LowerSaturationLimit=Lower_saturation_limit
  Out1 : Outport
  wires:
  In1/1 -> Ki/1, Kp/1
  Kp/1 -> Sum12/2
  Ki/1 -> integrator/1
  integrator/1 -> Sum12/1
  Saturation2/1 -> Out1/1
  Sum12/1 -> Saturation2/1

== system M4B11_modified_AGC_PI/Generator1/Machine Equations /Interface ==
  delta : Inport
  Vgxy : Inport  Port=2
  Eqd'' : Inport  Port=3
  Bx : Fcn  Expr=1/Xq11+(1/Xd11-1/Xq11)*sin(u(1))*sin(u(1))
  By : Fcn  Expr=-1/Xq11-(1/Xd11-1/Xq11)*cos(u(1))*cos(u(1))
  Gx : Fcn  Expr=(1/Xd11-1/Xq11)*sin(u(1))*cos(u(1))
  Gy : Fcn  Expr=(1/Xq11-1/Xd11)*sin(u(1))*cos(u(1))
  Igx1 : Fcn  Expr=sin(u(1))*u(2)/Xd11-cos(u(1))*u(3)/Xq11
  Igy1 : Fcn  Expr=-cos(u(1))*u(2)/Xd11-sin(u(1))*u(3)/Xq11
  Mux{1..3,5} (4 alike) : Mux  Inputs=2
  Mux4 : Mux
  Scope1 : Scope
      settings: ActiveDisplayYMinimum=0.73198  ActiveDisplayYMaximum=0.74189  DataLoggingVariableName=ScopeData5
  Vdg : Fcn  Expr=u(1)*sin(u(3))-u(2)*cos(u(3))
  Vqg : Fcn  Expr=u(1)*cos(u(3))+u(2)*sin(u(3))
  Vdqg : Outport
  Igxy1 : Outport  Port=2
  GBxy : Outport  Port=3
  wires:
  Vgxy/1 -> Mux1/1
  delta/1 -> By/1, Bx/1, Gy/1, Gx/1, Mux1/2, Mux5/1
  Eqd''/1 -> Mux5/2
  Vdg/1 -> Scope1/1, Mux2/1
  Vqg/1 -> Mux2/2
  Mux2/1 -> Vdqg/1
  Igx1/1 -> Mux3/1
  Igy1/1 -> Mux3/2
  Mux3/1 -> Igxy1/1
  Gx/1 -> Mux4/1
  Gy/1 -> Mux4/2
  Bx/1 -> Mux4/3
  By/1 -> Mux4/4
  Mux4/1 -> GBxy/1
  Mux1/1 -> Vdg/1, Vqg/1
  Mux5/1 -> Igx1/1, Igy1/1

== system M4B11_modified_AGC_PI/Generator1/Machine Equations /Transient Equations ==
  note: Eq
  Idqg : Inport
  Ef : Inport  Port=2
  Trip : Inport  Port=3
  Constant{1..4} (4 alike) : Constant  Value=0
  Ed' : Integrator  InitialCondition=Ed10
  Ed‘’ : Integrator  InitialCondition=Ed110
  Eq' : Integrator  InitialCondition=Eq10
  Eq‘’ : Integrator  InitialCondition=Eq110
  Fcn1 : Fcn  Expr=u(3)-(Xd1-Xd11)*u(1)-u(4)
  Fcn2 : Fcn  Expr=(Xq-Xq1)*u(2)-u(3)
  Fcn3 : Fcn  Expr=-u(1)+(Xq1-Xq11)*u(3)+u(4)
  Fcn7 : Fcn  Expr=u(3)+(Xd-Xd1)*u(1)
  Gain1 : Gain  Gain=1/Td10  SaturateOnIntegerOverflow=on  OutDataTypeStr=Inherit: Same as input  ParamDataTypeStr=Inherit: Same as input
  Gain2 : Gain  Gain=1/Tq0  SaturateOnIntegerOverflow=on  OutDataTypeStr=Inherit: Same as input  ParamDataTypeStr=Inherit: Same as input
  Gain3 : Gain  Gain=1/Td0  SaturateOnIntegerOverflow=on  OutDataTypeStr=Inherit: Same as input  ParamDataTypeStr=Inherit: Same as input
  Gain4 : Gain  Gain=1/Tq10  SaturateOnIntegerOverflow=on  OutDataTypeStr=Inherit: Same as input  ParamDataTypeStr=Inherit: Same as input
  Mux{1..4,6} (5 alike) : Mux  Inputs=2
  Sum1 : Sum  Inputs=|+-  SaturateOnIntegerOverflow=on
  Sum2 : Sum  Inputs=|++  SaturateOnIntegerOverflow=on
  Sum3 : Sum  Inputs=|++  SaturateOnIntegerOverflow=on
  Switch{1..8} (8 alike) : Switch  Criteria=u2 ~= 0  Threshold=0.5  InputSameDT=off
  Eqd'' : Outport
  wires:
  Gain3/1 -> Sum2/2, Switch5/3
  Sum1/1 -> Gain3/1
  Mux6/1 -> Fcn7/1, Mux1/1
  Fcn7/1 -> Sum1/2
  Idqg/1 -> Mux2/1, Mux6/1
  Ef/1 -> Sum1/1
  Gain1/1 -> Sum2/1
  Fcn1/1 -> Gain1/1
  Mux1/1 -> Fcn1/1
  Mux2/1 -> Fcn2/1, Mux4/2
  Fcn2/1 -> Gain2/1
  Gain2/1 -> Switch2/3, Sum3/2
  Mux3/1 -> Eqd''/1
  Gain4/1 -> Sum3/1
  Fcn3/1 -> Gain4/1
  Mux4/1 -> Fcn3/1
  Constant1/1 -> Switch2/1, Switch3/1
  Switch2/1 -> Ed'/1
  Ed'/1 -> Switch3/3
  Switch3/1 -> Mux2/2
  Trip/1 -> [Trip]
  [Trip] -> Switch3/2, Switch2/2
  Sum3/1 -> Switch1/3
  Switch1/1 -> Ed‘’/1
  Ed‘’/1 -> Switch4/3
  Switch4/1 -> Mux4/1, Mux3/2
  Constant2/1 -> Switch1/1, Switch4/1
  [Trip] -> Switch4/2, Switch1/2
  Switch5/1 -> Eq'/1
  Eq'/1 -> Switch6/3
  Switch6/1 -> Mux6/2
  Constant3/1 -> Switch6/1, Switch5/1
  [Trip] -> Switch6/2, Switch5/2
  Sum2/1 -> Switch7/3
  Switch7/1 -> Eq‘’/1
  Switch8/1 -> Mux1/2, Mux3/1
  Eq‘’/1 -> Switch8/3
  [Trip] -> Switch8/2, Switch7/2
  Constant4/1 -> Switch7/1, Switch8/1

== system M4B11_modified_AGC_PI/Generator2/Machine Equations /Interface ==
  delta : Inport
  Vgxy : Inport  Port=2
  Eqd'' : Inport  Port=3
  Bx : Fcn  Expr=1/Xq11+(1/Xd11-1/Xq11)*sin(u(1))*sin(u(1))
  By : Fcn  Expr=-1/Xq11-(1/Xd11-1/Xq11)*cos(u(1))*cos(u(1))
  Gx : Fcn  Expr=(1/Xd11-1/Xq11)*sin(u(1))*cos(u(1))
  Gy : Fcn  Expr=(1/Xq11-1/Xd11)*sin(u(1))*cos(u(1))
  Igx1 : Fcn  Expr=sin(u(1))*u(2)/Xd11-cos(u(1))*u(3)/Xq11
  Igy1 : Fcn  Expr=-cos(u(1))*u(2)/Xd11-sin(u(1))*u(3)/Xq11
  Mux{1..3,5} (4 alike) : Mux  Inputs=2
  Mux4 : Mux
  Scope1 : Scope
      settings: ActiveDisplayYMinimum=0.73198  ActiveDisplayYMaximum=0.74189  DataLoggingVariableName=ScopeData5
  Vdg : Fcn  Expr=u(1)*sin(u(3))-u(2)*cos(u(3))
  Vqg : Fcn  Expr=u(1)*cos(u(3))+u(2)*sin(u(3))
  Vdqg : Outport
  Igxy1 : Outport  Port=2
  GBxy : Outport  Port=3
  wires:
  Vgxy/1 -> Mux1/1
  delta/1 -> By/1, Bx/1, Gy/1, Gx/1, Mux1/2, Mux5/1
  Eqd''/1 -> Mux5/2
  Vdg/1 -> Scope1/1, Mux2/1
  Vqg/1 -> Mux2/2
  Mux2/1 -> Vdqg/1
  Igx1/1 -> Mux3/1
  Igy1/1 -> Mux3/2
  Mux3/1 -> Igxy1/1
  Gx/1 -> Mux4/1
  Gy/1 -> Mux4/2
  Bx/1 -> Mux4/3
  By/1 -> Mux4/4
  Mux4/1 -> GBxy/1
  Mux1/1 -> Vdg/1, Vqg/1
  Mux5/1 -> Igx1/1, Igy1/1

== system M4B11_modified_AGC_PI/Generator2/Machine Equations /Transient Equations ==
  note: Eq
  Idqg : Inport
  Ef : Inport  Port=2
  Trip : Inport  Port=3
  Constant{1..4} (4 alike) : Constant  Value=0
  Ed' : Integrator  InitialCondition=Ed10
  Ed‘’ : Integrator  InitialCondition=Ed110
  Eq' : Integrator  InitialCondition=Eq10
  Eq‘’ : Integrator  InitialCondition=Eq110
  Fcn1 : Fcn  Expr=u(3)-(Xd1-Xd11)*u(1)-u(4)
  Fcn2 : Fcn  Expr=(Xq-Xq1)*u(2)-u(3)
  Fcn3 : Fcn  Expr=-u(1)+(Xq1-Xq11)*u(3)+u(4)
  Fcn7 : Fcn  Expr=u(3)+(Xd-Xd1)*u(1)
  Gain1 : Gain  Gain=1/Td10  SaturateOnIntegerOverflow=on  OutDataTypeStr=Inherit: Same as input  ParamDataTypeStr=Inherit: Same as input
  Gain2 : Gain  Gain=1/Tq0  SaturateOnIntegerOverflow=on  OutDataTypeStr=Inherit: Same as input  ParamDataTypeStr=Inherit: Same as input
  Gain3 : Gain  Gain=1/Td0  SaturateOnIntegerOverflow=on  OutDataTypeStr=Inherit: Same as input  ParamDataTypeStr=Inherit: Same as input
  Gain4 : Gain  Gain=1/Tq10  SaturateOnIntegerOverflow=on  OutDataTypeStr=Inherit: Same as input  ParamDataTypeStr=Inherit: Same as input
  Mux{1..4,6} (5 alike) : Mux  Inputs=2
  Sum1 : Sum  Inputs=|+-  SaturateOnIntegerOverflow=on
  Sum2 : Sum  Inputs=|++  SaturateOnIntegerOverflow=on
  Sum3 : Sum  Inputs=|++  SaturateOnIntegerOverflow=on
  Switch{1..8} (8 alike) : Switch  Criteria=u2 ~= 0  Threshold=0.5  InputSameDT=off
  Eqd'' : Outport
  wires:
  Gain3/1 -> Sum2/2, Switch5/3
  Sum1/1 -> Gain3/1
  Mux6/1 -> Fcn7/1, Mux1/1
  Fcn7/1 -> Sum1/2
  Idqg/1 -> Mux2/1, Mux6/1
  Ef/1 -> Sum1/1
  Gain1/1 -> Sum2/1
  Fcn1/1 -> Gain1/1
  Mux1/1 -> Fcn1/1
  Mux2/1 -> Fcn2/1, Mux4/2
  Fcn2/1 -> Gain2/1
  Gain2/1 -> Switch2/3, Sum3/2
  Mux3/1 -> Eqd''/1
  Gain4/1 -> Sum3/1
  Fcn3/1 -> Gain4/1
  Mux4/1 -> Fcn3/1
  Constant1/1 -> Switch2/1, Switch3/1
  Switch2/1 -> Ed'/1
  Ed'/1 -> Switch3/3
  Switch3/1 -> Mux2/2
  Trip/1 -> [Trip]
  [Trip] -> Switch3/2, Switch2/2
  Sum3/1 -> Switch1/3
  Switch1/1 -> Ed‘’/1
  Ed‘’/1 -> Switch4/3
  Switch4/1 -> Mux4/1, Mux3/2
  Constant2/1 -> Switch1/1, Switch4/1
  [Trip] -> Switch4/2, Switch1/2
  Switch5/1 -> Eq'/1
  Eq'/1 -> Switch6/3
  Switch6/1 -> Mux6/2
  Constant3/1 -> Switch6/1, Switch5/1
  [Trip] -> Switch6/2, Switch5/2
  Sum2/1 -> Switch7/3
  Switch7/1 -> Eq‘’/1
  Switch8/1 -> Mux1/2, Mux3/1
  Eq‘’/1 -> Switch8/3
  [Trip] -> Switch8/2, Switch7/2
  Constant4/1 -> Switch7/1, Switch8/1

== system M4B11_modified_AGC_PI/Generator3/Machine Equations /Interface ==
  delta : Inport
  Vgxy : Inport  Port=2
  Eqd'' : Inport  Port=3
  Bx : Fcn  Expr=1/Xq11+(1/Xd11-1/Xq11)*sin(u(1))*sin(u(1))
  By : Fcn  Expr=-1/Xq11-(1/Xd11-1/Xq11)*cos(u(1))*cos(u(1))
  Gx : Fcn  Expr=(1/Xd11-1/Xq11)*sin(u(1))*cos(u(1))
  Gy : Fcn  Expr=(1/Xq11-1/Xd11)*sin(u(1))*cos(u(1))
  Igx1 : Fcn  Expr=sin(u(1))*u(2)/Xd11-cos(u(1))*u(3)/Xq11
  Igy1 : Fcn  Expr=-cos(u(1))*u(2)/Xd11-sin(u(1))*u(3)/Xq11
  Mux{1..3,5} (4 alike) : Mux  Inputs=2
  Mux4 : Mux
  Scope1 : Scope
      settings: ActiveDisplayYMinimum=0.73198  ActiveDisplayYMaximum=0.74189  DataLoggingVariableName=ScopeData5
  Vdg : Fcn  Expr=u(1)*sin(u(3))-u(2)*cos(u(3))
  Vqg : Fcn  Expr=u(1)*cos(u(3))+u(2)*sin(u(3))
  Vdqg : Outport
  Igxy1 : Outport  Port=2
  GBxy : Outport  Port=3
  wires:
  Vgxy/1 -> Mux1/1
  delta/1 -> By/1, Bx/1, Gy/1, Gx/1, Mux1/2, Mux5/1
  Eqd''/1 -> Mux5/2
  Vdg/1 -> Scope1/1, Mux2/1
  Vqg/1 -> Mux2/2
  Mux2/1 -> Vdqg/1
  Igx1/1 -> Mux3/1
  Igy1/1 -> Mux3/2
  Mux3/1 -> Igxy1/1
  Gx/1 -> Mux4/1
  Gy/1 -> Mux4/2
  Bx/1 -> Mux4/3
  By/1 -> Mux4/4
  Mux4/1 -> GBxy/1
  Mux1/1 -> Vdg/1, Vqg/1
  Mux5/1 -> Igx1/1, Igy1/1

== system M4B11_modified_AGC_PI/Generator3/Machine Equations /Transient Equations ==
  note: Eq
  Idqg : Inport
  Ef : Inport  Port=2
  Trip : Inport  Port=3
  Constant{1..4} (4 alike) : Constant  Value=0
  Ed' : Integrator  InitialCondition=Ed10
  Ed‘’ : Integrator  InitialCondition=Ed110
  Eq' : Integrator  InitialCondition=Eq10
  Eq‘’ : Integrator  InitialCondition=Eq110
  Fcn1 : Fcn  Expr=u(3)-(Xd1-Xd11)*u(1)-u(4)
  Fcn2 : Fcn  Expr=(Xq-Xq1)*u(2)-u(3)
  Fcn3 : Fcn  Expr=-u(1)+(Xq1-Xq11)*u(3)+u(4)
  Fcn7 : Fcn  Expr=u(3)+(Xd-Xd1)*u(1)
  Gain1 : Gain  Gain=1/Td10  SaturateOnIntegerOverflow=on  OutDataTypeStr=Inherit: Same as input  ParamDataTypeStr=Inherit: Same as input
  Gain2 : Gain  Gain=1/Tq0  SaturateOnIntegerOverflow=on  OutDataTypeStr=Inherit: Same as input  ParamDataTypeStr=Inherit: Same as input
  Gain3 : Gain  Gain=1/Td0  SaturateOnIntegerOverflow=on  OutDataTypeStr=Inherit: Same as input  ParamDataTypeStr=Inherit: Same as input
  Gain4 : Gain  Gain=1/Tq10  SaturateOnIntegerOverflow=on  OutDataTypeStr=Inherit: Same as input  ParamDataTypeStr=Inherit: Same as input
  Mux{1..4,6} (5 alike) : Mux  Inputs=2
  Sum1 : Sum  Inputs=|+-  SaturateOnIntegerOverflow=on
  Sum2 : Sum  Inputs=|++  SaturateOnIntegerOverflow=on
  Sum3 : Sum  Inputs=|++  SaturateOnIntegerOverflow=on
  Switch{1..8} (8 alike) : Switch  Criteria=u2 ~= 0  Threshold=0.5  InputSameDT=off
  Eqd'' : Outport
  wires:
  Gain3/1 -> Sum2/2, Switch5/3
  Sum1/1 -> Gain3/1
  Mux6/1 -> Fcn7/1, Mux1/1
  Fcn7/1 -> Sum1/2
  Idqg/1 -> Mux2/1, Mux6/1
  Ef/1 -> Sum1/1
  Gain1/1 -> Sum2/1
  Fcn1/1 -> Gain1/1
  Mux1/1 -> Fcn1/1
  Mux2/1 -> Fcn2/1, Mux4/2
  Fcn2/1 -> Gain2/1
  Gain2/1 -> Switch2/3, Sum3/2
  Mux3/1 -> Eqd''/1
  Gain4/1 -> Sum3/1
  Fcn3/1 -> Gain4/1
  Mux4/1 -> Fcn3/1
  Constant1/1 -> Switch2/1, Switch3/1
  Switch2/1 -> Ed'/1
  Ed'/1 -> Switch3/3
  Switch3/1 -> Mux2/2
  Trip/1 -> [Trip]
  [Trip] -> Switch3/2, Switch2/2
  Sum3/1 -> Switch1/3
  Switch1/1 -> Ed‘’/1
  Ed‘’/1 -> Switch4/3
  Switch4/1 -> Mux4/1, Mux3/2
  Constant2/1 -> Switch1/1, Switch4/1
  [Trip] -> Switch4/2, Switch1/2
  Switch5/1 -> Eq'/1
  Eq'/1 -> Switch6/3
  Switch6/1 -> Mux6/2
  Constant3/1 -> Switch6/1, Switch5/1
  [Trip] -> Switch6/2, Switch5/2
  Sum2/1 -> Switch7/3
  Switch7/1 -> Eq‘’/1
  Switch8/1 -> Mux1/2, Mux3/1
  Eq‘’/1 -> Switch8/3
  [Trip] -> Switch8/2, Switch7/2
  Constant4/1 -> Switch7/1, Switch8/1

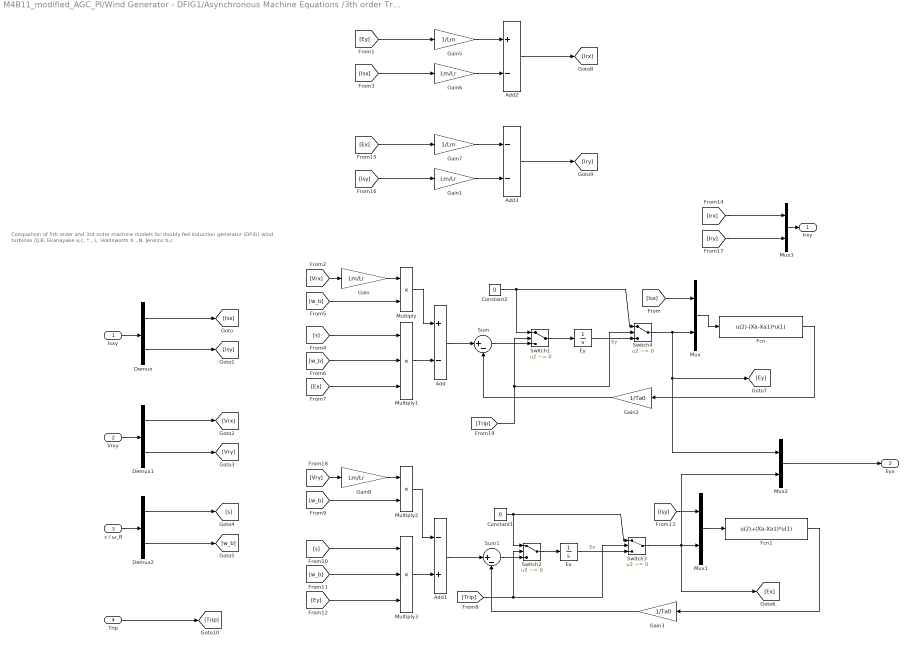
== system M4B11_modified_AGC_PI/Wind Generator - DFIG1/Asynchronous Machine Equations /3th order Transient Equations ==
  note: Comparison of 5th order and 3rd order machine models for doubly fed induction generator (DFIG) wind turbines
      | //J.B. Ekanayake a,c, * , L. Holdsworth b , N. Jenkins b,c
  Isxy : Inport
  Vrxy : Inport  Port=2
  s / ω_B : Inport  Port=3
  Trip : Inport  Port=4
  Add : Sum  Inputs=+-
  Add1 : Sum  Inputs=-+
  Add2 : Sum  Inputs=+-
  Add3 : Sum  Inputs=--
  Constant1 : Constant  Value=0
  Constant2 : Constant  Value=0
  Demux : Demux  Outputs=2
  Demux1 : Demux  Outputs=2
  Demux2 : Demux  Outputs=2
  Ex : Integrator  InitialCondition=Ex0
  Ey : Integrator  InitialCondition=Ey0
  Fcn : Fcn  Expr=u(2)-(Xa-Xa1)*u(1)
  Fcn1 : Fcn  Expr=u(2)+(Xa-Xa1)*u(1)
  Gain{,1,6,8} (4 alike) : Gain  Gain=Lm/Lr
  Gain2 : Gain  Gain=1/Ta0
  Gain3 : Gain  Gain=1/Ta0
  Gain5 : Gain  Gain=1/Lm
  Gain7 : Gain  Gain=1/Lm
  Multiply : Product
  Multiply1 : Product  Inputs=3
  Multiply2 : Product
  Multiply3 : Product  Inputs=3
  Mux{,1..3} (4 alike) : Mux  Inputs=2
  Sum : Sum  Inputs=|+-
  Sum1 : Sum  Inputs=|+-
  Switch{1..4} (4 alike) : Switch  Criteria=u2 ~= 0  Threshold=0.5  InputSameDT=off
  Irxy : Outport
  Eyx : Outport  Port=2
  wires:
  [Trip] -> Switch4/2, Switch1/2
  Constant2/1 -> Switch4/1, Switch1/1
  Switch4/1 -> Mux/2, [Ey], Mux2/1
  Ey/1 -> Switch4/3  "Ey"
  Switch1/1 -> Ey/1
  Sum/1 -> Switch1/3
  [Trip] -> Switch2/2, Switch3/2
  Constant1/1 -> Switch3/1, Switch2/1
  Switch3/1 -> Mux1/2, [Ex], Mux2/2
  Ex/1 -> Switch3/3  "Ex"
  Sum1/1 -> Switch2/3
  Switch2/1 -> Ex/1
  Trip/1 -> [Trip]
  [Vry] -> Gain8/1
  Gain8/1 -> Multiply2/1
  Gain/1 -> Multiply/1
  Add3/1 -> [Iry]
  [Isy] -> Gain1/1
  Add2/1 -> [Irx]
  Gain1/1 -> Add3/2
  [Isx] -> Gain6/1
  [Ey] -> Gain5/1
  Gain7/1 -> Add3/1
  [Ex] -> Gain7/1
  Gain6/1 -> Add2/2
  Gain5/1 -> Add2/1
  [Irx] -> Mux3/1
  [Iry] -> Mux3/2
  Mux3/1 -> Irxy/1
  Gain2/1 -> Sum/2
  Gain3/1 -> Sum1/2
  Mux2/1 -> Eyx/1
  Fcn1/1 -> Gain3/1
  Mux1/1 -> Fcn1/1
  [Isy] -> Mux1/1
  Add1/1 -> Sum1/1
  Multiply2/1 -> Add1/1
  Multiply3/1 -> Add1/2
  [s] -> Multiply3/1
  [Ey] -> Multiply3/3
  [w_b] -> Multiply3/2
  [w_b] -> Multiply2/2
  Multiply1/1 -> Add/2
  Add/1 -> Sum/1
  Multiply/1 -> Add/1
  Fcn/1 -> Gain2/1
  Mux/1 -> Fcn/1
  [Isx] -> Mux/1
  [Ex] -> Multiply1/3
  [w_b] -> Multiply1/2
  [s] -> Multiply1/1
  [w_b] -> Multiply/2
  [Vrx] -> Gain/1
  Demux1/2 -> [Vry]
  Demux1/1 -> [Vrx]
  Demux2/2 -> [w_b]
  Demux2/1 -> [s]
  s / ω_B/1 -> Demux2/1
  Vrxy/1 -> Demux1/1
  Isxy/1 -> Demux/1
  Demux/2 -> [Isy]
  Demux/1 -> [Isx]

== system M4B11_modified_AGC_PI/Wind Generator - DFIG1/Asynchronous Machine Equations /Interface ==
  delta : Inport
  Eqd : Inport  Port=2
  Add2 : Sum
  Add3 : Sum
  Bx : Constant  Value=Xa1/( Rs^2+Xa1^2 )
  By : Constant  Value=-Xa1/( Rs^2+Xa1^2 )
  Demux1 : Demux  Outputs=2
  Fcn : Fcn  Expr=(Rs*cos(u(1))+Xa1*sin(u(1))) / (Rs^2+Xa1^2)
  Fcn1 : Fcn  Expr=(Rs*cos(u(1))+Xa1*sin(u(1))) / (Rs^2+Xa1^2)
  Fcn2 : Fcn  Expr=(-Rs*sin(u(1))+Xa1*cos(u(1))) / (Rs^2+Xa1^2)
  Fcn3 : Fcn  Expr=(Rs*sin(u(1))-Xa1*cos(u(1))) / (Rs^2+Xa1^2)
  Gx : Constant  Value=Rs/( Rs^2+Xa1^2 )
  Gy : Constant  Value=Rs/( Rs^2+Xa1^2 )
  Mux3 : Mux  Inputs=2
  Mux4 : Mux
  Product{4..7} (4 alike) : Product
  Igxy1 : Outport
  GBxy : Outport  Port=2
  wires:
  Gx/1 -> Mux4/1
  [gx] -> Product4/1
  [Eq] -> Product5/1
  Product7/1 -> Add3/2
  Product4/1 -> Add2/1
  Product5/1 -> Add2/2
  Add3/1 -> [I1y]
  Product6/1 -> Add3/1
  [Eq] -> Product7/1
  [gy] -> Product7/2
  [bx] -> Product5/2
  Add2/1 -> [I1x]
  [Ed] -> Product6/2
  [Ed] -> Product4/2
  [by] -> Product6/1
  Fcn3/1 -> [by]
  Fcn2/1 -> [bx]
  Fcn1/1 -> [gy]
  Fcn/1 -> [gx]
  [delta] -> Fcn/1, Fcn3/1, Fcn2/1, Fcn1/1
  Demux1/2 -> [Ed]
  Demux1/1 -> [Eq]
  Mux4/1 -> GBxy/1
  By/1 -> Mux4/4
  Bx/1 -> Mux4/3
  Gy/1 -> Mux4/2
  Mux3/1 -> Igxy1/1
  [I1y] -> Mux3/2
  [I1x] -> Mux3/1
  Eqd/1 -> Demux1/1
  delta/1 -> [delta]

== system M4B11_modified_AGC_PI/Wind Generator - DFIG1/Rotor Side Converter control/Power Control ==
  note: $P_s^{ref}=2*(0.5000*\omega_r^2+0.0500*\omega_r+0.1200)$
  wr : Inport
  0-inf1 : Saturate  UpperLimit=inf  LowerLimit=0
  Tracking Curve5 : Fcn  Expr=1.162*u(1)^2
  Ps_ref : Outport
  wires:
  Tracking Curve5/1 -> Ps_ref/1
  0-inf1/1 -> Tracking Curve5/1
  wr/1 -> 0-inf1/1

== system M4B11_modified_AGC_PI/Wind Generator - DFIG1/Wind Turbine/Subsystem ==
  wind speed : Inport
  generator speed : Inport  Port=2
  Pitch angle (deg) : Inport  Port=3
  1/cp_nom : Gain  Gain=1/cp_nom  SaturateOnIntegerOverflow=on  OutDataTypeStr=Inherit: Same as input  ParamDataTypeStr=Inherit: Same as input
  Avoid division by zero : Saturate  UpperLimit=1e6  LowerLimit=1e-6
  "Avoid division by zero " : Saturate  UpperLimit=1e6  LowerLimit=1e-6
  Fcn : Fcn  Expr=1/(1/(u[1]+0.08*u[2])-0.035/(u[2]^3+1))
  Fcn1 : Fcn  Expr=c1*(c2/u[2]-c3*u[3]-c4)*exp(-c5/u[2])+c6*u[1]
  Gain : Gain  Gain=-1  SaturateOnIntegerOverflow=on  OutDataTypeStr=Inherit: Same as input  ParamDataTypeStr=Inherit: Same as input
  Mux : Mux  Inputs=2
  Mux1 : Mux  Inputs=3
  Product : Product  Inputs=/*  SaturateOnIntegerOverflow=on  OutDataTypeStr=Inherit: Same as first input
  "Product " : Product  SaturateOnIntegerOverflow=on  OutDataTypeStr=Inherit: Same as first input
  Product1 : Product  Inputs=*/  InputSameDT=on  SaturateOnIntegerOverflow=on  OutDataTypeStr=Inherit: Same as first input
  Saturation1 : Saturate  UpperLimit=inf  LowerLimit=1e-6
  lambda_nom : Gain  Gain=lambda_nom  SaturateOnIntegerOverflow=on  OutDataTypeStr=Inherit: Same as input  ParamDataTypeStr=Inherit: Same as input
  pu->pu : Gain  Gain=P_wind_base*Pnom/Pelec_base  SaturateOnIntegerOverflow=on  OutDataTypeStr=Inherit: Same as input  ParamDataTypeStr=Inherit: Same as input
  wind_speed^3 : Fcn  Expr=u(1)^3
  Tm : Outport
  wires:
  Pitch angle (deg)/1 -> Mux/2, Mux1/3
  Saturation1/1 -> Mux/1, Mux1/1
  Fcn1/1 -> 1/cp_nom/1
  Mux1/1 -> Fcn1/1
  Mux/1 -> Fcn/1
  Fcn/1 -> Mux1/2  "lambda_i"
  Gain/1 -> Tm/1
  Product1/1 -> Gain/1
  "Product "/1 -> pu->pu/1  "Pm_pu"
  lambda_nom/1 -> Saturation1/1
  generator speed/1 -> Avoid division by zero/1, Product/2
  "Avoid division by zero "/1 -> Product/1
  pu->pu/1 -> Product1/1
  Product/1 -> lambda_nom/1
  Avoid division by zero/1 -> Product1/2
  wind_speed^3/1 -> "Product "/1  "Pwind_pu"
  1/cp_nom/1 -> "Product "/2  "cp_pu"
  wind speed/1 -> "Avoid division by zero "/1, wind_speed^3/1  "wind_speed_pu"
